simulink model "DFT"  (R2017b)
settings: Solver=FixedStepDiscrete  StartTime=0.0  StopTime=simulationTime  RelTol=1e-3
PreLoadFcn:
  | DFT_init
undefined symbols (not defined in the file): jsin, nDistances, nRecurrences, nRecurrencesMax, oversamplingFactor, phaseIncrement, sampleTime
libraries: hdlsllib x6, dspsigops x3, simulink x1
settings Model: DataTypeOverride=Off  Creator=pnowodzi  LastModifiedBy=pnowodzi
settings DataIOCC: ExternalInput=currentSamples syncRecurrence syncAnalysis  LimitDataPoints=on  LoadExternalInput=on  SaveTime=off
settings OptimizationCC: BlockReduction=off  ConditionallyExecuteInputs=off  DefaultParameterBehavior=Inlined  LifeSpan=inf
settings DebuggingCC: AlgebraicLoopMsg=error  SingleTaskRateTransMsg=error  AllowSymbolicDim=off  StrictBusMsg=ErrorOnBusTreatedAsVector  SFUnexpectedBacktrackingDiag=warning  SFNoUnconditionalDefaultTransitionDiag=warning  SFExecutionAtInitializationDiag=none
settings HardwareCC: ProdBitPerPointer=32  ProdBitPerSizeT=32  ProdBitPerPtrDiffT=32  ProdLargestAtomicFloat=None  ProdIntDivRoundTo=Undefined  ProdEndianess=Unspecified  ProdWordSize=32  ProdHWDeviceType=ASIC/FPGA->ASIC/FPGA  ProdEqTarget=off
settings CodeAppCC: StateflowObjectComments=on
settings GRTTargetCC: TargetLangStandard=C89/C90 (ANSI)  GeneratePreprocessorConditionals=Disable all
settings ConfigComp: CovScope=ReferencedModels  CovMetricSettings=dw  CovHtmlReporting=on  CovSaveCumulativeToWorkspaceVar=on  CovSaveSingleToWorkspaceVar=on  CovExternalEMLEnable=off  CovSFcnEnable=off

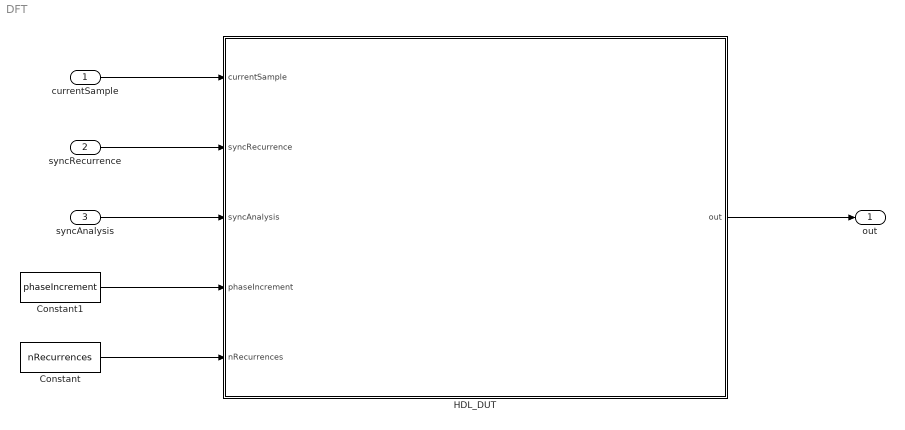
== system DFT ==
  currentSample : Inport  OutDataTypeStr=DTsample  SampleTime=sampleTime  Interpolate=off
      settings: SignalType=complex
  "syncRecurrence " : Inport  Port=2  OutDataTypeStr=boolean  SampleTime=sampleTime  Interpolate=off
  syncAnalysis : Inport  Port=3  OutDataTypeStr=boolean  SampleTime=sampleTime  Interpolate=off
  Constant : Constant  Value=nRecurrences  OutDataTypeStr=fixdt(0,10,0)  SampleTime=sampleTime
  Constant1 : Constant  Value=phaseIncrement  OutDataTypeStr=DTPhaseIncrement  SampleTime=sampleTime
  HDL_DUT : Subsystem
  out : Outport
  wires:
  currentSample/1 -> HDL_DUT/1(currentSample)
  "syncRecurrence "/1 -> HDL_DUT/2("syncRecurrence ")
  syncAnalysis/1 -> HDL_DUT/3(syncAnalysis)
  Constant1/1 -> HDL_DUT/4(phaseIncrement)
  Constant/1 -> HDL_DUT/5(nRecurrences)
  HDL_DUT/1(out) -> out/1

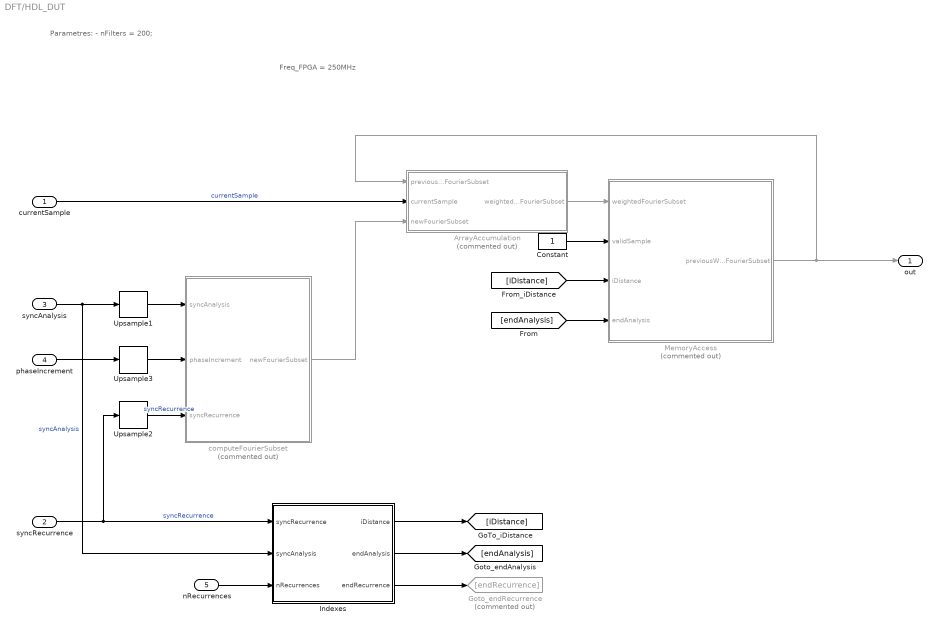
== system DFT/HDL_DUT ==
  note: Freq_FPGA = 250MHz
  note: Parametres:
      | - nFilters = 200;
  currentSample : Inport  OutDataTypeStr=DTsample  SampleTime=sampleTime
      settings: SignalType=complex
  "syncRecurrence " : Inport  Port=2  OutDataTypeStr=boolean
  syncAnalysis : Inport  Port=3  OutDataTypeStr=boolean
  phaseIncrement : Inport  Port=4  OutDataTypeStr=DTPhaseIncrement
  nRecurrences : Inport  Port=5  OutDataTypeStr=fixdt(0,10,0)
  ArrayAccumulation : Subsystem  Commented=on
  Constant : Constant  OutDataTypeStr=boolean  SampleTime=-1
  Goto_endRecurrence : Goto  Commented=on  GotoTag=endRecurrence
  Indexes : Subsystem
  MemoryAccess : Subsystem  Commented=on
  Upsample1 : dspsigops/Upsample  N=oversamplingFactor  phase=0  RateOptions=Allow multirate processing  ic=0  mode=Unused parameter value
  Upsample2 : dspsigops/Upsample  N=oversamplingFactor  phase=0  RateOptions=Allow multirate processing  ic=0  mode=Unused parameter value
  Upsample3 : dspsigops/Upsample  N=oversamplingFactor  phase=0  RateOptions=Allow multirate processing  ic=0  mode=Unused parameter value
  computeFourierSubset : Subsystem  Commented=on
  out : Outport
  wires:
  phaseIncrement/1 -> Upsample3/1
  syncAnalysis/1 -> Upsample1/1, Indexes/2(syncAnalysis)  "syncAnalysis"
  currentSample/1 -> ArrayAccumulation/2(currentSample)  "currentSample"
  MemoryAccess/1(previousWeightedFourierSubset) -> out/1, ArrayAccumulation/1(previousWeightedFourierSubset)
  computeFourierSubset/1(newFourierSubset) -> ArrayAccumulation/3(newFourierSubset)
  ArrayAccumulation/1(weightedFourierSubset) -> MemoryAccess/1(weightedFourierSubset)
  "syncRecurrence "/1 -> Indexes/1(syncRecurrence), Upsample2/1  "syncRecurrence"
  Indexes/1(iDistance) -> [iDistance]
  nRecurrences/1 -> Indexes/3(nRecurrences)
  Indexes/3(endRecurrence) -> Goto_endRecurrence/1
  Indexes/2(endAnalysis) -> [endAnalysis]
  Upsample1/1 -> computeFourierSubset/1(syncAnalysis)
  Upsample3/1 -> computeFourierSubset/2(phaseIncrement)
  Upsample2/1 -> computeFourierSubset/3(syncRecurrence)  "syncRecurrence"
  [iDistance] -> MemoryAccess/3(iDistance)
  [endAnalysis] -> MemoryAccess/4(endAnalysis)
  Constant/1 -> MemoryAccess/2(validSample)

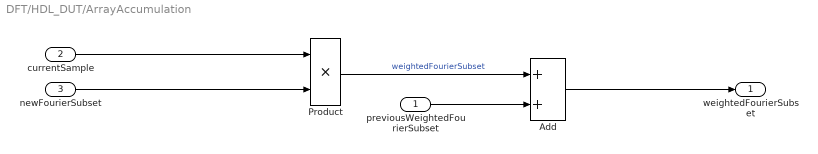
== system DFT/HDL_DUT/ArrayAccumulation ==
  previousWeightedFourierSubset : Inport
  currentSample : Inport  Port=2
  newFourierSubset : Inport  Port=3
  Add : Sum
  Product : Product
  weightedFourierSubset : Outport
  wires:
  newFourierSubset/1 -> Product/2
  Product/1 -> Add/1  "weightedFourierSubset"
  previousWeightedFourierSubset/1 -> Add/2
  Add/1 -> weightedFourierSubset/1
  currentSample/1 -> Product/1

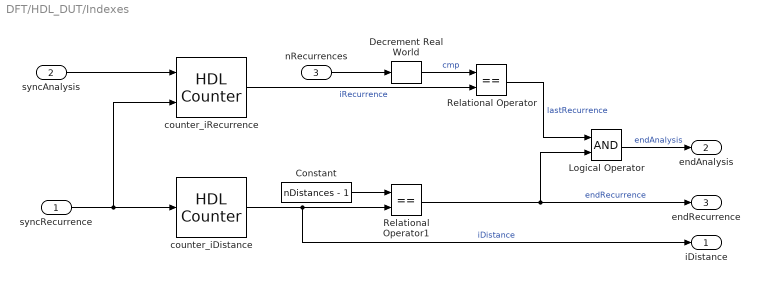
== system DFT/HDL_DUT/Indexes ==
  syncRecurrence : Inport
  syncAnalysis : Inport  Port=2
  nRecurrences : Inport  Port=3
  Constant : Constant  Value=nDistances - 1  SampleTime=-1
  Decrement Real World : simulink/Additional Math & Discrete/Additional Math: Increment - Decrement/Decrement Real World
      settings: SourceProductName=Simulink  SourceProductBaseCode=SL
  Logical Operator : Logic  AllPortsSameDT=off  OutDataTypeStr=boolean
  Relational Operator : RelationalOperator  Operator===  OutDataTypeStr=boolean  RndMeth=Nearest
  Relational Operator1 : RelationalOperator  Operator===  OutDataTypeStr=boolean  RndMeth=Nearest
  counter_iDistance : hdlsllib/Sources/HDL Counter  CountType=Free running  CountInit=0  CountStep=1  CountMax=25  CountFromType=Initial value  CountFrom=0  CountResetPort=on  CountLoadPort=off  CountEnbPort=off  CountDirPort=off  CountDataType=Unsigned  CountWordLen=ceil(log2(nDistances))  CountFracLen=0  CountSampTime=1
      settings: SourceProductBaseCode=HD
  counter_iRecurrence : hdlsllib/Sources/HDL Counter  CountType=Free running  CountInit=0  CountStep=1  CountMax=25  CountFromType=Initial value  CountFrom=0  CountResetPort=on  CountLoadPort=off  CountEnbPort=on  CountDirPort=off  CountDataType=Unsigned  CountWordLen=ceil(log2(nRecurrencesMax))  CountFracLen=0  CountSampTime=1
      settings: SourceProductBaseCode=HD
  iDistance : Outport
  endAnalysis : Outport  Port=2
  endRecurrence : Outport  Port=3
  wires:
  counter_iDistance/1 -> Relational Operator1/2, iDistance/1  "iDistance"
  syncAnalysis/1 -> counter_iRecurrence/1
  counter_iRecurrence/1 -> Relational Operator/2  "iRecurrence"
  syncRecurrence/1 -> counter_iDistance/1, counter_iRecurrence/2
  Relational Operator/1 -> Logical Operator/1  "lastRecurrence"
  nRecurrences/1 -> Decrement Real World/1
  Relational Operator1/1 -> endRecurrence/1, Logical Operator/2  "endRecurrence"
  Constant/1 -> Relational Operator1/1
  Decrement Real World/1 -> Relational Operator/1  "cmp"
  Logical Operator/1 -> endAnalysis/1  "endAnalysis"

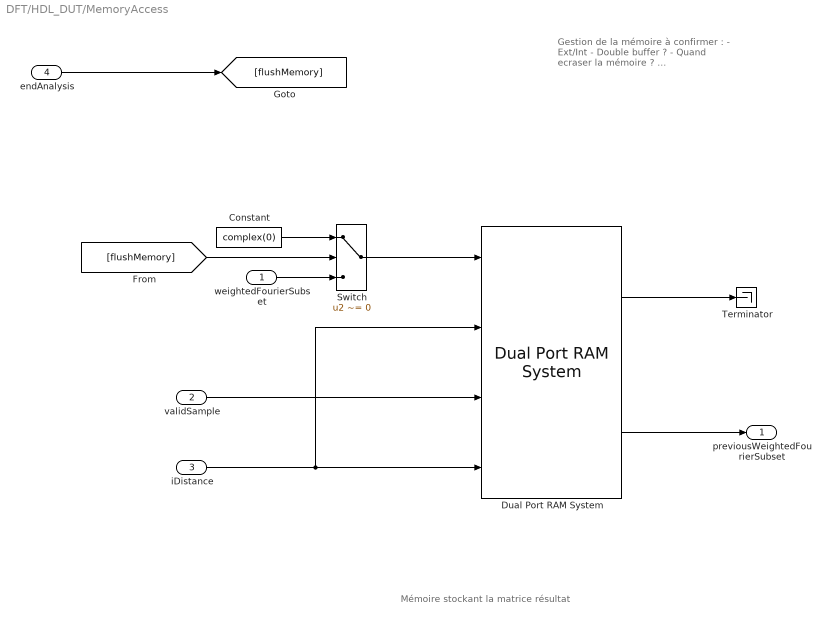
== system DFT/HDL_DUT/MemoryAccess ==
  note: Gestion de la mémoire à confirmer :
      |
      | - Ext/Int
      | - Double buffer ?
      | - Quand ecraser la mémoire ?
      | ...
  note: Mémoire stockant la matrice résultat
  weightedFourierSubset : Inport
  validSample : Inport  Port=2
  iDistance : Inport  Port=3
  endAnalysis : Inport  Port=4
  Constant : Constant  Value=complex(0)  SampleTime=-1
  Dual Port RAM System : hdlsllib/HDL RAMs/Dual Port RAM System  RAMType=Dual port  WriteOutputValue=New data  RAMInitialValue=0  SimulateUsing=Code generation
      settings: SourceProductName=HDL Coder  SourceProductBaseCode=HD
  Switch : Switch  Criteria=u2 ~= 0
  Terminator : Terminator
  previousWeightedFourierSubset : Outport
  wires:
  Dual Port RAM System/2 -> previousWeightedFourierSubset/1
  validSample/1 -> Dual Port RAM System/3
  iDistance/1 -> Dual Port RAM System/4, Dual Port RAM System/2
  Switch/1 -> Dual Port RAM System/1
  Constant/1 -> Switch/1
  endAnalysis/1 -> [flushMemory]
  weightedFourierSubset/1 -> Switch/3
  [flushMemory] -> Switch/2
  Dual Port RAM System/1 -> Terminator/1

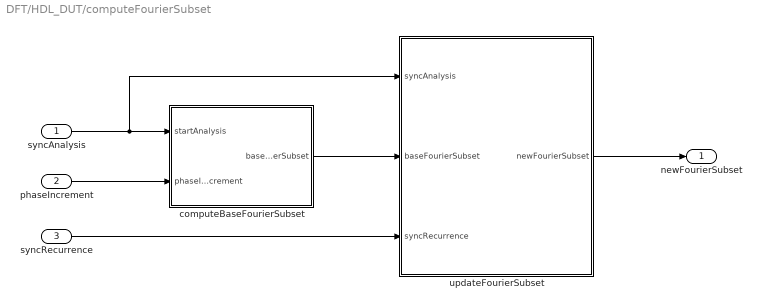
== system DFT/HDL_DUT/computeFourierSubset ==
  syncAnalysis : Inport
  phaseIncrement : Inport  Port=2
  syncRecurrence : Inport  Port=3
  computeBaseFourierSubset : Subsystem
  updateFourierSubset : Subsystem
  newFourierSubset : Outport
  wires:
  computeBaseFourierSubset/1(baseFourierSubset) -> updateFourierSubset/2(baseFourierSubset)
  syncAnalysis/1 -> updateFourierSubset/1(syncAnalysis), computeBaseFourierSubset/1(startAnalysis)
  updateFourierSubset/1(newFourierSubset) -> newFourierSubset/1
  syncRecurrence/1 -> updateFourierSubset/3(syncRecurrence)
  phaseIncrement/1 -> computeBaseFourierSubset/2(phaseIncrement)

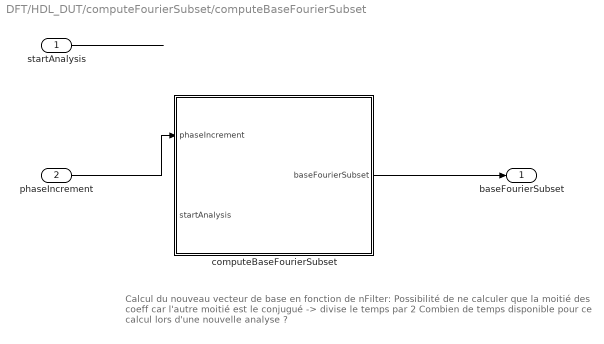
== system DFT/HDL_DUT/computeFourierSubset/computeBaseFourierSubset ==
  note: Calcul du nouveau vecteur de base  en fonction de nFilter:
      | Possibilité de ne calculer que la moitié des coeff car l'autre moitié est le conjugué -> divise le temps par 2
      |
      |
      | Combien de temps disponible pour ce calcul lors d'une nouvelle analyse ?
  startAnalysis : Inport
  phaseIncrement : Inport  Port=2
  computeBaseFourierSubset : Subsystem
  baseFourierSubset : Outport
  wires:
  computeBaseFourierSubset/1(baseFourierSubset) -> baseFourierSubset/1
  startAnalysis/1 -> ?
  phaseIncrement/1 -> computeBaseFourierSubset/1(phaseIncrement)

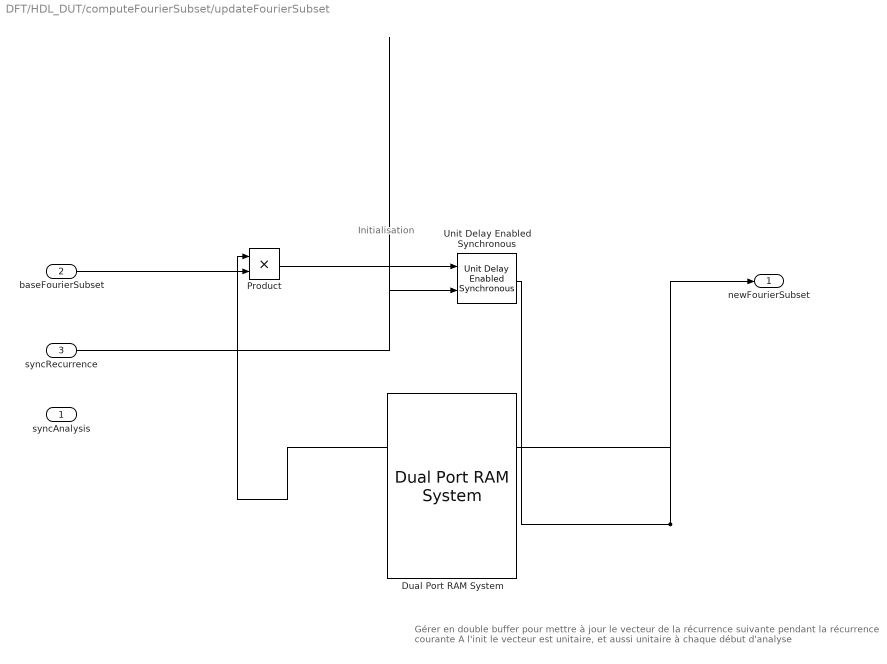
== system DFT/HDL_DUT/computeFourierSubset/updateFourierSubset ==
  note: Gérer en double buffer pour mettre à jour le vecteur de la récurrence suivante pendant la récurrence courante
      |
      | A l'init le vecteur est unitaire, et aussi unitaire à chaque début d'analyse
  note: Initialisation
  syncAnalysis : Inport
  baseFourierSubset : Inport  Port=2
  syncRecurrence : Inport  Port=3
  Dual Port RAM System : hdlsllib/HDL RAMs/Dual Port RAM System  RAMType=Dual port  WriteOutputValue=New data  RAMInitialValue=0  SimulateUsing=Code generation
      settings: SourceProductName=HDL Coder  SourceProductBaseCode=HD
  Product : Product
  Unit Delay Enabled Synchronous : hdlsllib/Discrete/Unit Delay Enabled Synchronous  InitialCondition=0.0  SampleTime=-1
      settings: SourceProductName=HDL Coder  SourceProductBaseCode=HD
  newFourierSubset : Outport
  wires:
  Product/1 -> Unit Delay Enabled Synchronous/1
  baseFourierSubset/1 -> Product/2
  Unit Delay Enabled Synchronous/1 -> Product/1, newFourierSubset/1
  syncRecurrence/1 -> Unit Delay Enabled Synchronous/2

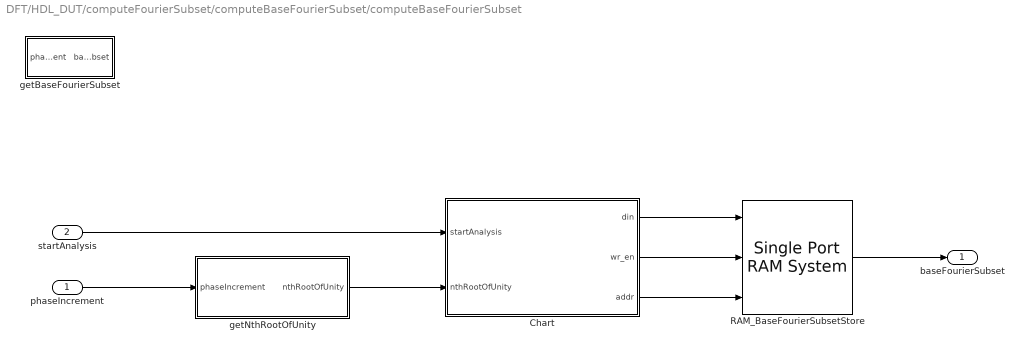
== system DFT/HDL_DUT/computeFourierSubset/computeBaseFourierSubset/computeBaseFourierSubset ==
  phaseIncrement : Inport
  startAnalysis : Inport  Port=2
  Chart : Stateflow chart  TreatAsAtomicUnit=on
  RAM_BaseFourierSubsetStore : hdlsllib/HDL RAMs/Single Port RAM System  RAMType=Single port  WriteOutputValue=New data  RAMInitialValue=0  SimulateUsing=Code generation
      settings: SourceProductName=HDL Coder  SourceProductBaseCode=HD
  getBaseFourierSubset : MATLAB Function  TreatAsAtomicUnit=on
  getNthRootOfUnity : Subsystem
  baseFourierSubset : Outport
  wires:
  RAM_BaseFourierSubsetStore/1 -> baseFourierSubset/1
  phaseIncrement/1 -> getNthRootOfUnity/1(phaseIncrement)
  getNthRootOfUnity/1(nthRootOfUnity) -> Chart/2(nthRootOfUnity)
  Chart/1(din) -> RAM_BaseFourierSubsetStore/1
  Chart/3(addr) -> RAM_BaseFourierSubsetStore/3
  Chart/2(wr_en) -> RAM_BaseFourierSubsetStore/2
  startAnalysis/1 -> Chart/1(startAnalysis)

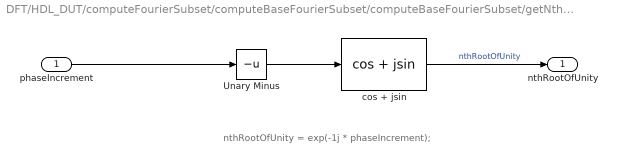
== system DFT/HDL_DUT/computeFourierSubset/computeBaseFourierSubset/computeBaseFourierSubset/getNthRootOfUnity ==
  note: nthRootOfUnity = exp(-1j * phaseIncrement);
  phaseIncrement : Inport
  Unary Minus : UnaryMinus
  cos + jsin : Trigonometry  Operator=cos + jsin
  nthRootOfUnity : Outport
  wires:
  phaseIncrement/1 -> Unary Minus/1
  Unary Minus/1 -> cos + jsin/1
  cos + jsin/1 -> nthRootOfUnity/1  "nthRootOfUnity"

== matlab function DFT/HDL_DUT/computeFourierSubset/computeBaseFourierSubset/computeBaseFourierSubset/getBaseFourierSubset ==
  data: phaseIncrement input; baseFourierSubset output; nFilters parameter
function baseFourierSubset = getBaseFourierSubset(phaseIncrement, nFilters)
% phaseIncrement =     2 * pi / nRecurrences

    baseFourierSubset    = complex(zeros(nFilters, 1));
    nthRootOfUnity   = exp(-1j * phaseIncrement);
    iCenterElement = floor(nFilters / 2) + 1;
    baseFourierSubset(iCenterElement) = 1;
    for iElement = 1:iCenterElement - 1
        baseFourierSubset(iCenterElement + iElement) = baseFourierSubset(iCenterElement + iElement - 1) * nthRootOfUnity;
        baseFourierSubset(iCenterElement - iElement) = conj(baseFourierSubset(iCenterElement + iElement));
    end
end

== stateflow chart DFT/HDL_DUT/computeFourierSubset/computeBaseFourierSubset/computeBaseFourierSubset/Chart ==
  settings: executeAtInitialization=1
  data: startAnalysis input; nthRootOfUnity input; din output double; wr_en output double; addr output double
